simulink model "Switch_data_inspector"  (R2024b)
settings: Solver=FixedStepAuto  StartTime=0.0  StopTime=10.0  FixedStep=0.0001  RelTol=1e-3
settings Model: Creator=abdal  LastModifiedBy=abdal

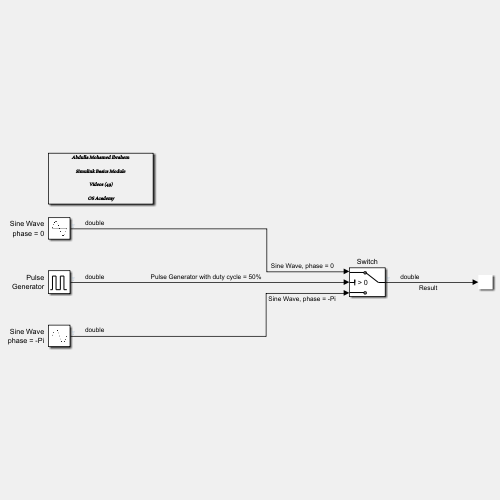
[thumbnail: Simulink's stored preview of the top-level diagram]
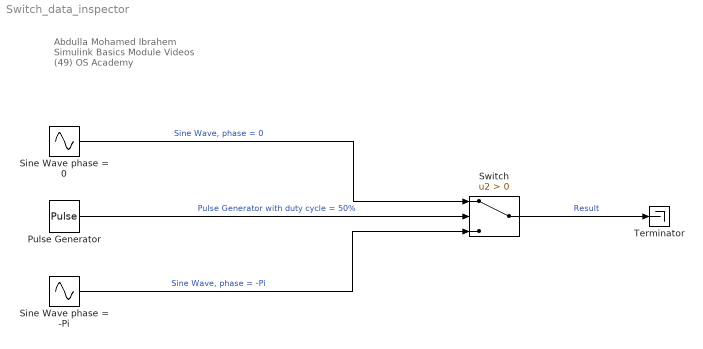
== system Switch_data_inspector ==
  note: Abdulla Mohamed Ibrahem
      | Simulink Basics Module
      | Videos (49)
      | OS Academy
  Pulse Generator : DiscretePulseGenerator  PulseType=Time based  Period=1  PulseWidth=50
  Sine Wave phase = -Pi : Sin  Phase=-1*pi  SampleTime=0
  Sine Wave phase = 0 : Sin  SampleTime=0
  Switch : Switch  Criteria=u2 > Threshold  SaturateOnIntegerOverflow=off  InputSameDT=off
  Terminator : Terminator
  wires:
  Pulse Generator/1 -> Switch/2  "Pulse Generator with duty cycle = 50%"
  Sine Wave phase = 0/1 -> Switch/1  "Sine Wave, phase = 0"
  Sine Wave phase = -Pi/1 -> Switch/3  "Sine Wave, phase = -Pi"
  Switch/1 -> Terminator/1  "Result"
